simulink model "model"  (R2014b)
settings: Solver=ode23s  StartTime=0.0  StopTime=100  FixedStep=5e-5  RelTol=1e-3
values from neighbouring files (symbols this model uses):
  Fc = 1    [main.m]
  Fs = 1.5    [main.m]
  Ki = 4    [main.m]
  Kp = 3    [main.m]
  Kv = 6    [main.m]
  sigma0 = 1e5    (= 100000)    [main.m]
  sigma1 = sqrt(1e5)    [main.m]
  sigma2 = 0.4    [main.m]
  vs = 0.001    [main.m]
settings Model: Creator=123  LastModifiedBy=123
settings DataIOCC: LimitDataPoints=off
settings DebuggingCC: MaxConsecutiveZCsMsg=none  SolverPrmCheckMsg=none

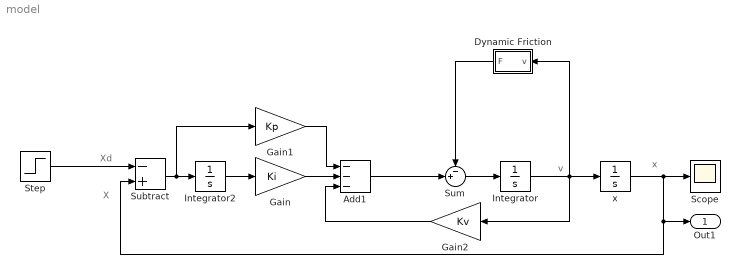
== system model ==
  note: X
  note: Xd
  note: x
  note: v
  Add1 : Sum  Inputs=---
  Dynamic Friction : Subsystem
  Gain : Gain  Gain=Ki
  Gain1 : Gain  Gain=Kp
  Gain2 : Gain  Gain=Kv
  Integrator : Integrator
  Integrator2 : Integrator
  Scope : Scope
      settings: ShowLegends=on  YMin=0  YMax=1.6  ScrollMode=on
  Step : Step  Time=0  SampleTime=0
  Subtract : Sum  Inputs=-+
  Sum : Sum  Inputs=-+|
  x : Integrator
  Out1 : Outport
  wires:
  Integrator/1 -> x/1, Gain2/1, Dynamic Friction/1(v)
  Dynamic Friction/1(F) -> Sum/1
  Sum/1 -> Integrator/1
  x/1 -> Subtract/2, Out1/1, Scope/1
  Subtract/1 -> Gain1/1, Integrator2/1
  Integrator2/1 -> Gain/1
  Step/1 -> Subtract/1
  Gain2/1 -> Add1/3
  Gain/1 -> Add1/2
  Gain1/1 -> Add1/1
  Add1/1 -> Sum/2

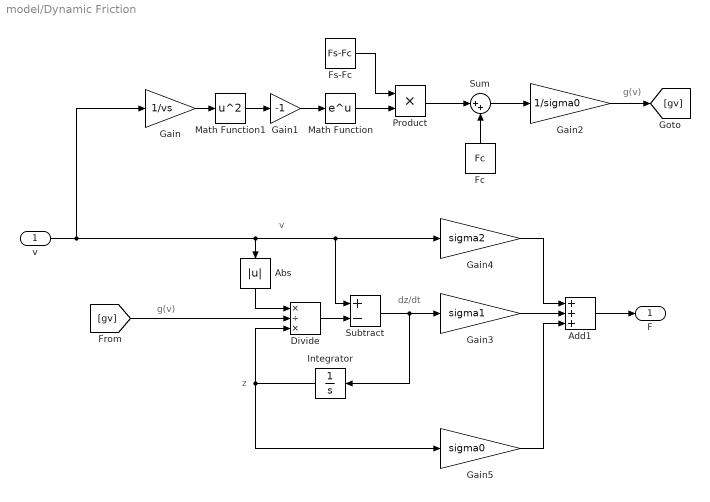
== system model/Dynamic Friction ==
  note: z
  note: g(v)
  note: v
  note: dz/dt
  note: g(v)
  v : Inport
  Abs : Abs
  Add1 : Sum  Inputs=+++
  Divide : Product  Inputs=*/*
  Fc : Constant  Value=Fc
  Fs-Fc : Constant  Value=Fs-Fc
  Gain : Gain  Gain=1/vs
  Gain1 : Gain  Gain=-1
  Gain2 : Gain  Gain=1/sigma0
  Gain3 : Gain  Gain=sigma1
  Gain4 : Gain  Gain=sigma2
  Gain5 : Gain  Gain=sigma0
  Integrator : Integrator
  Math Function : Math  SaturateOnIntegerOverflow=on
  Math Function1 : Math  Operator=square  SaturateOnIntegerOverflow=on
  Product : Product
  Subtract : Sum  Inputs=+-
  Sum : Sum  Inputs=|++
  F : Outport
  wires:
  Math Function/1 -> Product/2
  Product/1 -> Sum/1
  Fs-Fc/1 -> Product/1
  Divide/1 -> Subtract/2
  Math Function1/1 -> Gain1/1
  Gain/1 -> Math Function1/1
  Fc/1 -> Sum/2
  Sum/1 -> Gain2/1
  v/1 -> Subtract/1, Gain4/1, Abs/1, Gain/1
  Subtract/1 -> Integrator/1, Gain3/1
  Gain4/1 -> Add1/1
  Gain5/1 -> Add1/3
  Gain3/1 -> Add1/2
  Add1/1 -> F/1
  Gain1/1 -> Math Function/1
  Abs/1 -> Divide/1
  [gv] -> Divide/2
  Gain2/1 -> [gv]
  Integrator/1 -> Divide/3, Gain5/1
